simulink model "lpspi_master_slave_s32k11x"  (Simulink 9.0)
settings: Solver=FixedStepDiscrete  StartTime=0.0  StopTime=10.0  FixedStep=0.5  RelTol=1e-3  EnableMultiTasking=on
InitFcn:
  | mbd_s32k_consistency_checks(bdroot(gcs));
undefined symbols (not defined in the file): LQFP, thumb
libraries: mbd_s32k1xx_ec_toolbox x8, simulink x1
Description:
  | This demo shows how to use 2 instances of LPSPI (one master, one slave) to transfer data and trigger a subsystem
  | at TRANSFER END event.
  | 
  | HW requirements:
  |  - 1 S32K118 EVB
  | 
  | Please connect the following:
  | [Master: MOSI] B4 J2.4 - J1.11 D1 [Slave: MOSI]
  | [Master: MISO] B3 J2.5 - J1.6   E0 [Slave: MISO]
  | [Master: PCS0] B5 J2.3 - J1.8   E1 [Slave: PCS0]
  | [Master: SCK]   B2 J2.6 - J1.9  D0 [Slave: SCK]
  | 
  | Note: MOSI (Master Output Slave Input) <=> [Master] SOut - [Slave] SIn connection
  | 
  | Verification:
  |  - The GREEN LED should blink every 0.5s
  |  - You can open the FreeMASTER project (same name as the model) and you should see MOSI and MISO values
  |    Note: MOSI value should be MISO Value + 1 or +2, depending on the order of the blocks (in the code generation).
settings Model: Creator=NXP MBDT Team  LastModifiedBy=nxf35172
settings DataIOCC: ExternalInput=off  InitialState=off  LimitDataPoints=on  SaveOutput=off  SignalLogging=off  SaveTime=off
settings OptimizationCC: DefaultParameterBehavior=Inlined  LifeSpan=1
settings DebuggingCC: SolverPrmCheckMsg=warning  InheritedTsInSrcMsg=none  SingleTaskRateTransMsg=error  UnconnectedInputMsg=error  UnconnectedOutputMsg=error  UnconnectedLineMsg=error  AllowSymbolicDim=off  UnknownTsInhSupMsg=error  StateNameClashWarn=warning
settings HardwareCC: ProdLargestAtomicInteger=Long  ProdLargestAtomicFloat=Double  ProdIntDivRoundTo=Zero  ProdEndianess=LittleEndian  ProdHWDeviceType=ARM Compatible->ARM Cortex
settings SFSimCC: MATLABDynamicMemAlloc=off
settings RTWCC: SystemTargetFile=mbd_s32k.tlc  MakeCommand=mbd_s32k_make_rtw COPY_MDLREF_INCLUDES=0  TemplateMakefile=mbd_s32k.tmf  Description=Model Based Design Toolbox S32K14x Code Generation Target  GenerateReport=on  IncludeHyperlinkInReport=on  LaunchReport=on  GenerateTraceInfo=on  GenerateTraceReport=on  GenerateTraceReportSl=on  GenerateTraceReportSf=on  GenerateTraceReportEml=on
settings CodeAppCC: ForceParamTrailComments=on  IgnoreCustomStorageClasses=off  OperatorAnnotations=on  SimulinkDataObjDesc=on  SFDataObjDesc=on  MATLABFcnDesc=on  InsertBlockDesc=on  MATLABSourceComments=on
settings STFCustomTargetCC: CombineOutputUpdateFcns=on  ERTCustomFileBanners=on  SupportContinuousTime=off  SupportNonInlinedSFcns=off  RemoveResetFunc=on  MATLABClassNameForMDSCustomization=Simulink.SoftwareTarget.ERTCustomization  GRTInterface=off  SystemTargetFile=mbd_s32k14.tlc
settings ERTTargetCC: MultiwordLength=2048  ParMdlRefBuildCompliant=off  CompOptLevelCompliant=off  ConcurrentExecutionCompliant=off  ModelStepFunctionPrototypeControlCompliant=off  CPPClassGenCompliant=off  UseToolchainInfoCompliant=off  InlinedParameterPlacement=NonHierarchical  ERTSrcFileBannerTemplate=mbd_ert_code_template.cgt  ERTHdrFileBannerTemplate=mbd_ert_code_template.cgt  ERTDataSrcFileTemplate=mbd_ert_code_template.cgt  ERTDataHdrFileTemplate=mbd_ert_code_template.cgt  ERTCustomFileTemplate=example_file_process.tlc

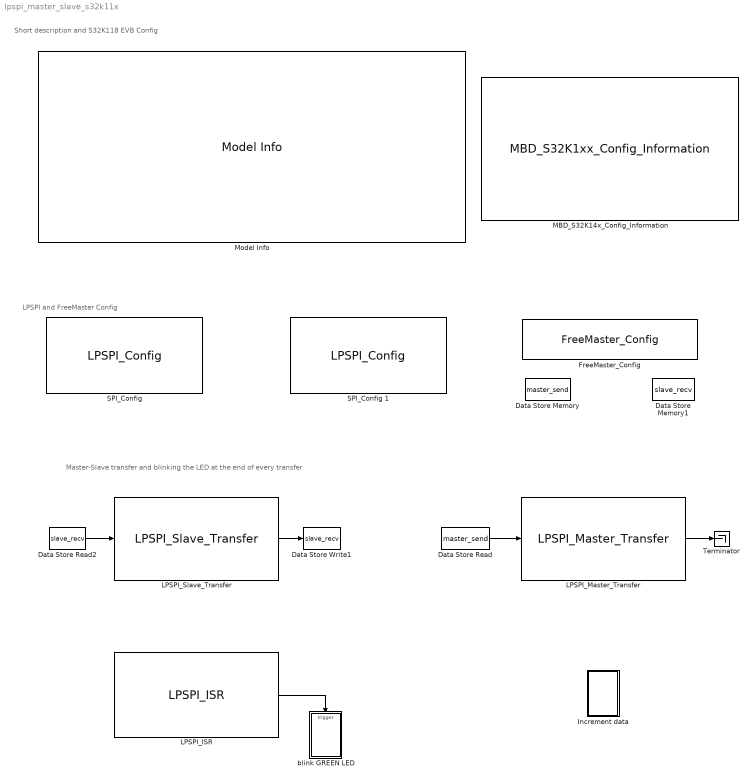
== system lpspi_master_slave_s32k11x ==
  note: Master-Slave transfer and blinking the LED at the end of every transfer
  note: LPSPI and FreeMaster Config
  note: Short description and S32K118 EVB Config
  Data Store Memory : DataStoreMemory  Priority=2  DataStoreName=master_send  ReadBeforeWriteMsg=warning  WriteAfterWriteMsg=warning  WriteAfterReadMsg=warning  InitialValue=2  ShowAdditionalParam=off  OutDataTypeStr=uint8
  Data Store Memory1 : DataStoreMemory  Priority=2  DataStoreName=slave_recv  ReadBeforeWriteMsg=warning  WriteAfterWriteMsg=warning  WriteAfterReadMsg=warning  ShowAdditionalParam=off  OutDataTypeStr=uint8
  Data Store Read : DataStoreRead  DataStoreName=master_send
  Data Store Read2 : DataStoreRead  Priority=1  DataStoreName=slave_recv
  Data Store Write1 : DataStoreWrite  DataStoreName=slave_recv
  FreeMaster_Config : mbd_s32k1xx_ec_toolbox/Utility Blocks/FreeMaster_Config  Priority=3  interface=LPUART0  baudrate=115200  rxd=PTB0: [LPUART0_RX | Receive]  txd=PTB1: [LPUART0_TX | Transmit]  mode=Short Interrupt  isr_prio=1  show_adv_opts=on  use_scope=on  max_scope_vars=8  use_recorder=on  max_rec_vars=8  rec_buff_size=1024  rec_timebase=0 seconds  comm_buffer_size_auto=on  comm_buffer_size=255  comm_rqueue_size_default=on  comm_rqueue_size=32
  Increment data : Subsystem
  LPSPI_ISR : mbd_s32k1xx_ec_toolbox/Communication Blocks/SPI Blocks/LPSPI_ISR  instanceNumber=0  isr_lvl=0  role=Master  transfer_end=on  spi_upd=on
  LPSPI_Master_Transfer : mbd_s32k1xx_ec_toolbox/Communication Blocks/SPI Blocks/LPSPI_Master_Transfer  Priority=4  instance=0  pcs=1  pcs_polarity=ActiveLow  xfermode=Non blocking  timeout=200  spi_upd=on
  LPSPI_Slave_Transfer : mbd_s32k1xx_ec_toolbox/Communication Blocks/SPI Blocks/LPSPI_Slave_Transfer  Priority=3  instance=1  pcs=0  pcs_polarity=ActiveLow  xfermode=Non blocking  timeout=200  spi_upd=on
  MBD_S32K14x_Config_Information : mbd_s32k1xx_ec_toolbox/MBD_S32K1xx_Config_Information  mbdt_ver=0  disp_str=|  config_params=[]  mcu_target_name=S32K118  mcu_target_package=48-LQFP  mcu_target_sram_size=25KB  mcu_system_clock_freq=40  mcu_xtal_freq=External 40  mcu_steptick_timer=LPIT Channel 0  mcu_steptick_prio=0  ds_import_enable=on  target_compiler=GCC  target_memory=FLASH  gcc_target_compile_opts=-mcpu=cortex-m0plus -mthumb -O1 -g -gstrict-dwarf  gcc_target_assemble_opts=-mcpu=cortex-m0plus -mthumb -g  gcc_target_link_opts=-mcpu=cortex-m0plus -mthumb  gcc_target_default_lcf=on  gcc_target_user_lcf=S32K118_25_flash.ld  ghs_target_compile_opts=-mcpu=cortexm0plus -mthumb -fsoft -Ogeneral -Wundef -Wimplicit-int -Wshadow -Wtrigraphs --no_commons --gnu_asm -gnu99 -gdwarf-2 -G  ghs_target_assemble_opts=-mcpu=cortexm0plus -mthumb -fsoft --gnu_asm  ghs_target_link_opts=-mcpu=cortexm0plus -mthumb -fsoft  ghs_target_default_lcf=off  ghs_target_user_lcf=S32K118_25_flash.ld  iar_target_compile_opts=--thumb -Ol -e --debug --dlib_config normal  iar_target_assemble_opts=--thumb  iar_target_link_opts=--no_exceptions --vfe --inline  iar_target_default_lcf=off  iar_target_user_lcf=S32K118_25_flash.icf  pil_download_enable=off  rbl_download_enable=on  rbl_start_delay=5000000  rbl_download_interface=OpenSDA  rbl_restart_request=off  rbl_com_port=Custom  rbl_com_port_custom=COM1  pil_download_rate=57600  pil_opensda_drive=Custom  pil_opensda_drive_custom=D  pil_uart_instance=0  pil_uart_rx=PTB0: [LPUART0_RX | Receive]  pil_uart_tx=PTB1: [LPUART0_TX | Transmit]  FTM_PWM_PcrCheckEnDis=on  FTM_Input_Edge_Inputs_PcrCheckEnDis=on  FTM_Dual_Edge_Inputs_PcrCheckEnDis=on  FTM_Quadrature_Inputs_PcrCheckEnDis=on  FTM_Hall_Sensor_Inputs_PcrCheckEnDis=on  LPTMR_PcrCheckEnDis=on  PIT_PcrCheckEnDis=on  RTC_PcrCheckEnDis=on  FlexCAN_PcrCheckEnDis=on  LIN_PcrCheckEnDis=on  FlexIO_PcrCheckEnDis=on  LPI2C_PcrCheckEnDis=on  LPSPI_PcrCheckEnDis=on  LPUART_PcrCheckEnDis=on  CMP_PcrCheckEnDis=on  GPIO_OutputPcrCheckEnDis=on  GPIO_InputPcrCheckEnDis=on  SBC_PcrCheckEnDis=on  AMMCLIB_PcrCheckEnDis=on  FM_PcrCheckEnDis=on  Profile_PcrCheckEnDis=on  ConfigParams_PcrCheckEnDis=on  ModelRef_PcrCheckEnDis=on  PDB0_PcrCheckEnDis=on  CSEc_PcrCheckEnDis=on  eDMA_PcrCheckEnDis=on  ADC_PcrCheckEnDis=on  WDOG_PcrCheckEnDis=on
      | Target : S32K144-64KB_SRAM
      | Package : 100-pin
      | System clock : 80 MHz
      | XTAL clock : External 8 MHz
      | Compiler : IAR
      | Target Type : FLASH
      | Download Code after build : off
      | Step Tick Interrupt Priority : 15
  Model Info : simulink/Model-Wide Utilities/Model Info  Frame=off  DisplayStringWithTags=|  HorizontalTextAlignment=Left  LeftAlignmentValue=0.02
      | Model Name: %<ModelName>
      | 
      | Description: %<Description>
  "SPI_Config " : mbd_s32k1xx_ec_toolbox/Communication Blocks/SPI Blocks/LPSPI_Config   Priority=2  InstanceNumber=0  Role=Master  BaudRate=50000  ShowAdvanced=on  sin=PTB3: [LPSPI0_SIN | LPSPI Serial Data Input]  sout=PTB4: [LPSPI0_SOUT | LPSPI Serial Data Output]  sck=PTB2: [LPSPI0_SCK | LPSPI Serial Clock I/O]  pcs0=None  pcs1=PTB5: [LPSPI0_PCS1 | Peripheral Chip Select 1]  pcs2=None  pcs3=not available  CPHA=0  CPOL=0  BitOrder=MSB first  TransferSize=8  WhichPCS=1  PCSPol=ActiveLow  ContinuousTransfer=off
  SPI_Config 1 : mbd_s32k1xx_ec_toolbox/Communication Blocks/SPI Blocks/LPSPI_Config   Priority=2  InstanceNumber=1  Role=Slave  BaudRate=100  ShowAdvanced=on  sin=PTD1: [LPSPI1_SIN | LPSPI Serial Data Input]  sout=PTD2: [LPSPI1_SOUT | LPSPI Serial Data Output]  sck=PTD0: [LPSPI1_SCK | LPSPI Serial Clock I/O]  pcs0=None  pcs1=None  pcs2=not available  pcs3=not available  CPHA=0  CPOL=0  BitOrder=MSB first  TransferSize=8  WhichPCS=0  PCSPol=ActiveLow  ContinuousTransfer=off
  Terminator : Terminator
  blink GREEN LED : Subsystem
  wires:
  Data Store Read/1 -> LPSPI_Master_Transfer/1
  LPSPI_Master_Transfer/1 -> Terminator/1
  Data Store Read2/1 -> LPSPI_Slave_Transfer/1
  LPSPI_Slave_Transfer/1 -> Data Store Write1/1
  LPSPI_ISR/1 -> blink GREEN LED/Trigger

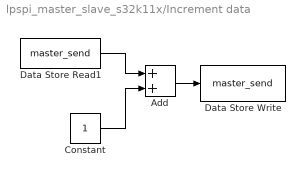
== system lpspi_master_slave_s32k11x/Increment data ==
  Add : Sum  Priority=3
  Constant : Constant  OutDataTypeStr=uint8
  Data Store Read1 : DataStoreRead  DataStoreName=master_send
  Data Store Write : DataStoreWrite  DataStoreName=master_send
  wires:
  Add/1 -> Data Store Write/1
  Data Store Read1/1 -> Add/1
  Constant/1 -> Add/2

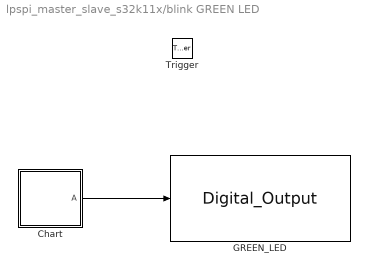
== system lpspi_master_slave_s32k11x/blink GREEN LED ==
  Trigger : TriggerPort  TriggerType=function-call  VariantControl=Variant  PortDimensions=1
  Chart : Stateflow chart  TreatAsAtomicUnit=on
  GREEN_LED : mbd_s32k1xx_ec_toolbox/GPIO Blocks/Digital_Output  gpio_pin=PTD15: [PTD15 | Port D I/O]  init_val=Low  drive_strength=Low
  wires:
  Chart/1(" A") -> GREEN_LED/1

== stateflow chart blink GREEN LED/Chart ==
  state A
  state A1
  (default) -> A
  A -> A1
  A1 -> A
  data: A output boolean [0..1]
